simulink model "ins_anello_C9R_HIL_candidate"  (R2026a)
settings: Solver=FixedStepAuto  FixedStep=0.004
undefined symbols (not defined in the file or in its folder): vehicle
settings Model: Creator=Usuario  LastModifiedBy=Edison Altamirano

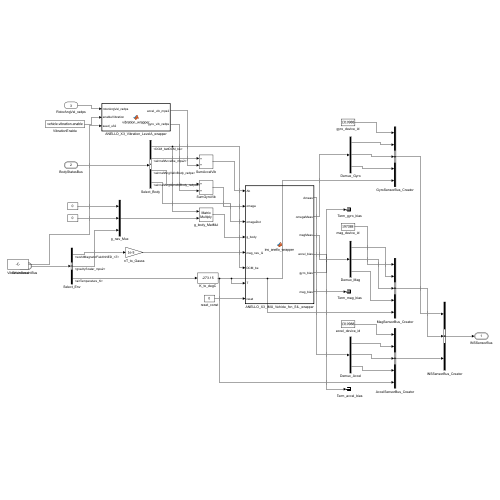
[thumbnail: Simulink's stored preview of the top-level diagram]
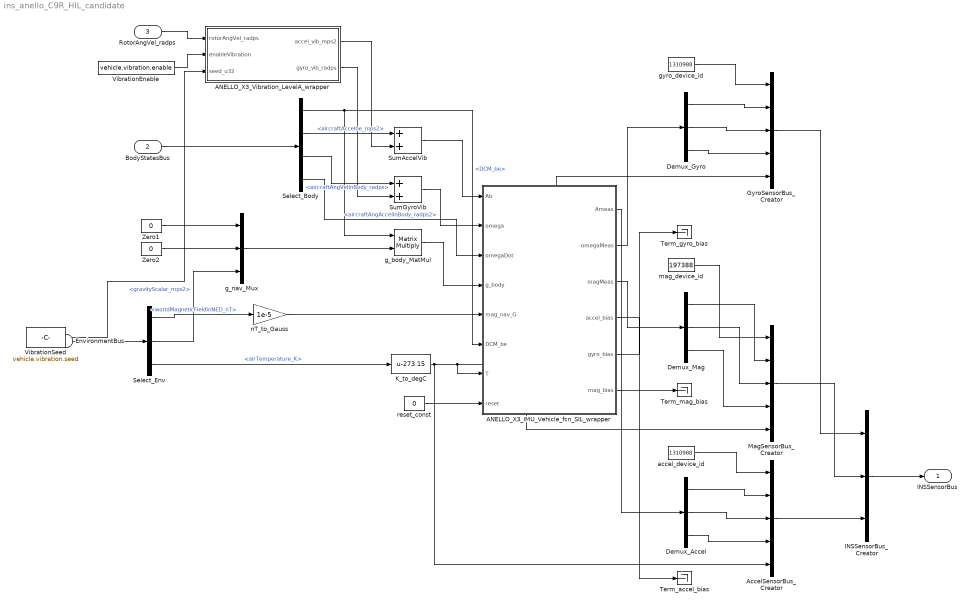
== system ins_anello_C9R_HIL_candidate ==
  EnvironmentBus : Inport  OutDataTypeStr=Bus: EnvironmentBus
  BodyStatesBus : Inport  Port=2  OutDataTypeStr=Bus: BodyStateBus
  RotorAngVel_radps : Inport  Port=3  PortDimensions=6
  ANELLO_X3_IMU_Vehicle_fcn_SIL_wrapper : MATLAB Function  TreatAsAtomicUnit=on
  ANELLO_X3_Vibration_LevelA_wrapper : MATLAB Function  TreatAsAtomicUnit=on
  AccelSensorBus_Creator : BusCreator  Inputs=5  OutDataTypeStr=Bus: AccelSensorBus
  Demux_Accel : Demux  Outputs=3
  Demux_Gyro : Demux  Outputs=3
  Demux_Mag : Demux  Outputs=3
  GyroSensorBus_Creator : BusCreator  Inputs=5  OutDataTypeStr=Bus: GyroSensorBus
  INSSensorBus_Creator : BusCreator  Inputs=3  OutDataTypeStr=Bus: INSSensorBus
  K_to_degC : Bias  Bias=-273.15  SaturateOnIntegerOverflow=off
  MagSensorBus_Creator : BusCreator  Inputs=5  OutDataTypeStr=Bus: MagSensorBus
  Select_Body : BusSelector  OutputSignals=DCM_be,aircraftAccelbe_mps2,aircraftAngVelInBody_radps,aircraftAngAccelInBody_radps2
  Select_Env : BusSelector  OutputSignals=EarthEnvironment.worldMagneticFieldInNED_nT,EarthEnvironment.gravityScalar_mps2,AirEnvironment.airTemperature_K
  SumAccelVib : Sum
  SumGyroVib : Sum
  Term_accel_bias : Terminator
  Term_gyro_bias : Terminator
  Term_mag_bias : Terminator
  VibrationEnable : Constant  Value=vehicle.vibration.enable
  VibrationSeed : Constant  Value=vehicle.vibration.seed
  Zero1 : Constant  Value=0
  Zero2 : Constant  Value=0
  accel_device_id : Constant  Value=1310988
  g_body_MatMul : Product  Multiplication=Matrix(*)
  g_nav_Mux : Mux  Inputs=3
  gyro_device_id : Constant  Value=1310988
  mag_device_id : Constant  Value=197388
  nT_to_Gauss : Gain  Gain=1e-5
  reset_const : Constant  Value=0
  INSSensorBus : Outport  OutDataTypeStr=Bus: INSSensorBus
  wires:
  BodyStatesBus/1 -> Select_Body/1
  VibrationEnable/1 -> ANELLO_X3_Vibration_LevelA_wrapper/2(enableVibration)
  EnvironmentBus/1 -> Select_Env/1
  RotorAngVel_radps/1 -> ANELLO_X3_Vibration_LevelA_wrapper/1(rotorAngVel_radps)
  Zero1/1 -> g_nav_Mux/1
  reset_const/1 -> ANELLO_X3_IMU_Vehicle_fcn_SIL_wrapper/8(reset)
  Select_Env/1 -> nT_to_Gauss/1  "<worldMagneticFieldInNED_nT>"
  SumAccelVib/1 -> ANELLO_X3_IMU_Vehicle_fcn_SIL_wrapper/1(Ab)
  Zero2/1 -> g_nav_Mux/2
  Select_Env/2 -> g_nav_Mux/3  "<gravityScalar_mps2>"
  Select_Env/3 -> K_to_degC/1  "<airTemperature_K>"
  ANELLO_X3_Vibration_LevelA_wrapper/1(accel_vib_mps2) -> SumAccelVib/2
  ANELLO_X3_IMU_Vehicle_fcn_SIL_wrapper/5(gyro_bias) -> Term_gyro_bias/1
  ANELLO_X3_Vibration_LevelA_wrapper/2(gyro_vib_radps) -> SumGyroVib/2
  Demux_Gyro/1 -> GyroSensorBus_Creator/2
  Select_Body/1 -> ANELLO_X3_IMU_Vehicle_fcn_SIL_wrapper/6(DCM_be), g_body_MatMul/1  "<DCM_be>"
  Demux_Gyro/2 -> GyroSensorBus_Creator/3
  Select_Body/2 -> SumAccelVib/1  "<aircraftAccelbe_mps2>"
  Select_Body/3 -> SumGyroVib/1  "<aircraftAngVelInBody_radps>"
  Select_Body/4 -> ANELLO_X3_IMU_Vehicle_fcn_SIL_wrapper/3(omegaDot)  "<aircraftAngAccelInBody_radps2>"
  g_nav_Mux/1 -> g_body_MatMul/2
  nT_to_Gauss/1 -> ANELLO_X3_IMU_Vehicle_fcn_SIL_wrapper/5(mag_nav_G)
  Demux_Mag/2 -> MagSensorBus_Creator/3
  SumGyroVib/1 -> ANELLO_X3_IMU_Vehicle_fcn_SIL_wrapper/2(omega)
  g_body_MatMul/1 -> ANELLO_X3_IMU_Vehicle_fcn_SIL_wrapper/4(g_body)
  K_to_degC/1 -> MagSensorBus_Creator/5, GyroSensorBus_Creator/5, ANELLO_X3_IMU_Vehicle_fcn_SIL_wrapper/7(T), AccelSensorBus_Creator/5
  Demux_Accel/1 -> AccelSensorBus_Creator/2
  ANELLO_X3_IMU_Vehicle_fcn_SIL_wrapper/1(Ameas) -> Demux_Accel/1
  ANELLO_X3_IMU_Vehicle_fcn_SIL_wrapper/2(omegaMeas) -> Demux_Gyro/1
  GyroSensorBus_Creator/1 -> INSSensorBus_Creator/1
  ANELLO_X3_IMU_Vehicle_fcn_SIL_wrapper/3(magMeas) -> Demux_Mag/1
  ANELLO_X3_IMU_Vehicle_fcn_SIL_wrapper/4(accel_bias) -> Term_accel_bias/1
  ANELLO_X3_IMU_Vehicle_fcn_SIL_wrapper/6(mag_bias) -> Term_mag_bias/1
  gyro_device_id/1 -> GyroSensorBus_Creator/1
  Demux_Gyro/3 -> GyroSensorBus_Creator/4
  mag_device_id/1 -> MagSensorBus_Creator/1
  Demux_Mag/1 -> MagSensorBus_Creator/2
  Demux_Mag/3 -> MagSensorBus_Creator/4
  accel_device_id/1 -> AccelSensorBus_Creator/1
  MagSensorBus_Creator/1 -> INSSensorBus_Creator/2
  Demux_Accel/2 -> AccelSensorBus_Creator/3
  Demux_Accel/3 -> AccelSensorBus_Creator/4
  AccelSensorBus_Creator/1 -> INSSensorBus_Creator/3
  INSSensorBus_Creator/1 -> INSSensorBus/1
  VibrationSeed/1 -> ANELLO_X3_Vibration_LevelA_wrapper/3(seed_u32)

== matlab function ins_anello_C9R_HIL_candidate/ANELLO_X3_Vibration_LevelA_wrapper ==
  data: rotorAngVel_radps input; accel_vib_mps2 output; enableVibration input; gyro_vib_radps output; seed_u32 input
function [accel_vib_mps2, gyro_vib_radps] = vibration_wrapper(rotorAngVel_radps, enableVibration, seed_u32)
%#codegen
[accel_vib_mps2, gyro_vib_radps] = C9R_gyrocoupling_ANELLO_X3_Vibration_LevelA_fcn(rotorAngVel_radps, enableVibration, seed_u32);
end

== matlab function ins_anello_C9R_HIL_candidate/ANELLO_X3_IMU_Vehicle_fcn_SIL_wrapper ==
  data: Ab input; Ameas output; omega input; omegaDot input; g_body input; mag_nav_G input; DCM_be input; T input; reset input; omegaMeas output; magMeas output; accel_bias output; gyro_bias output; mag_bias output
function [Ameas, omegaMeas, magMeas, accel_bias, gyro_bias, mag_bias] = ...
         ins_anello_wrapper(Ab, omega, omegaDot, g_body, mag_nav_G, DCM_be, T, reset)
%#codegen
R_bn_vec = DCM_be(:);
[Ameas, omegaMeas, magMeas, accel_bias, gyro_bias, mag_bias] = ...
    ANELLO_X3_IMU_Vehicle_fcn_SIL(Ab, omega, omegaDot, g_body, mag_nav_G, R_bn_vec, T, reset);
end
